simulink model "Controle_velocidade"  (R2021a)
settings: Solver=VariableStepAuto  StartTime=0.0  StopTime=10.0  RelTol=1e-3
values from neighbouring files (symbols this model uses):
  B = 0    [P1_script.m]    (also in simulacao1.m)
  J = 0.001    [P1_script.m]    (also in simulacao1.m = 0.00252)
  Kac = 1/Kpc    (= 0.0936205547599)    [P1_script.m]
  Kas = 1/Kps    (= 0.676014937262)    [P1_script.m]
  Kic = Ra*2*pi*Wcc    (= 1633.62817987)    [P1_script.m]
  Kis = J*(2*pi*Wcs)^2/(5*Kt)    (= 185.888948923)    [P1_script.m]
  Kpc = La*2*pi*Wcc    (= 10.6814150222)    [P1_script.m]
  Kps = J*2*pi*Wcs/Kt    (= 1.47925725436)    [P1_script.m]
  Kt = Te_rated/Ia_rated    (= 0.424752712124)    [P1_script.m]    (also in simulacao1.m)
  La = 1.7e-3    (= 0.0017)    [P1_script.m]    (also in simulacao1.m)
  Ra = 0.26    [P1_script.m]    (also in simulacao1.m)
settings Model: Creator=taylo  LastModifiedBy=taylo

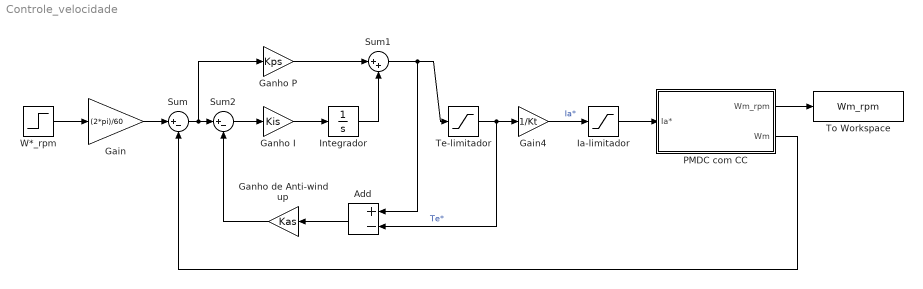
== system Controle_velocidade ==
  Add : Sum  Inputs=+-
  Gain : Gain  Gain=(2*pi)/60
  Gain4 : Gain  Gain=1/Kt
  Ganho I : Gain  Gain=Kis
  Ganho P : Gain  Gain=Kps
  Ganho de Anti-wind up : Gain  Gain=Kas
  Ia-limitador : Saturate
  Integrador : Integrator
  PMDC com CC : Subsystem
  Sum : Sum  Inputs=|+-
  Sum1 : Sum  Inputs=|++
  Sum2 : Sum  Inputs=|+-
  Te-limitador : Saturate
  To Workspace : ToWorkspace  VariableName=Wm_rpm  SaveFormat=Timeseries  SampleTime=-1
  W*_rpm : Step  SampleTime=0
  wires:
  Gain/1 -> Sum/1
  Integrador/1 -> Sum1/2
  Ganho P/1 -> Sum1/1
  Sum1/1 -> Add/1, Te-limitador/1
  Ganho I/1 -> Integrador/1
  Te-limitador/1 -> Add/2, Gain4/1  "Te*"
  Gain4/1 -> Ia-limitador/1  "Ia*"
  Ia-limitador/1 -> PMDC com CC/1(Ia*)
  Sum/1 -> Ganho P/1, Sum2/1
  Sum2/1 -> Ganho I/1
  Add/1 -> Ganho de Anti-wind up/1
  Ganho de Anti-wind up/1 -> Sum2/2
  W*_rpm/1 -> Gain/1
  PMDC com CC/1(Wm_rpm) -> To Workspace/1
  PMDC com CC/2(Wm) -> Sum/2

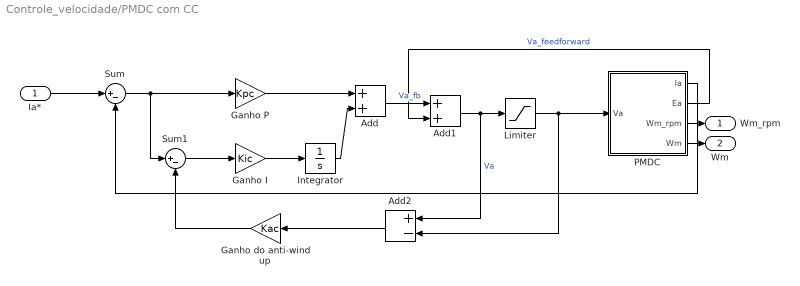
== system Controle_velocidade/PMDC com CC ==
  Ia* : Inport
  Add : Sum
  Add1 : Sum
  Add2 : Sum  Inputs=+-
  Ganho I : Gain  Gain=Kic
  Ganho P : Gain  Gain=Kpc
  Ganho do anti-wind up : Gain  Gain=Kac
  Integrator : Integrator
  Limiter : Saturate
  PMDC : Subsystem
  Sum : Sum  Inputs=|+-
  Sum1 : Sum  Inputs=|+-
  Wm_rpm : Outport
  Wm : Outport  Port=2
  wires:
  Sum/1 -> Sum1/1, Ganho P/1
  Integrator/1 -> Add/2
  Add1/1 -> Add2/1, Limiter/1  "Va"
  Limiter/1 -> Add2/2, PMDC/1(Va)
  Ganho P/1 -> Add/1
  PMDC/1(Ia) -> Sum/2
  Sum1/1 -> Ganho I/1
  Ganho do anti-wind up/1 -> Sum1/2
  Add2/1 -> Ganho do anti-wind up/1
  PMDC/2(Ea) -> Add1/2  "Va_feedforward"
  Add/1 -> Add1/1  "Va_fb"
  Ganho I/1 -> Integrator/1
  Ia*/1 -> Sum/1
  PMDC/4(Wm) -> Wm/1
  PMDC/3(Wm_rpm) -> Wm_rpm/1

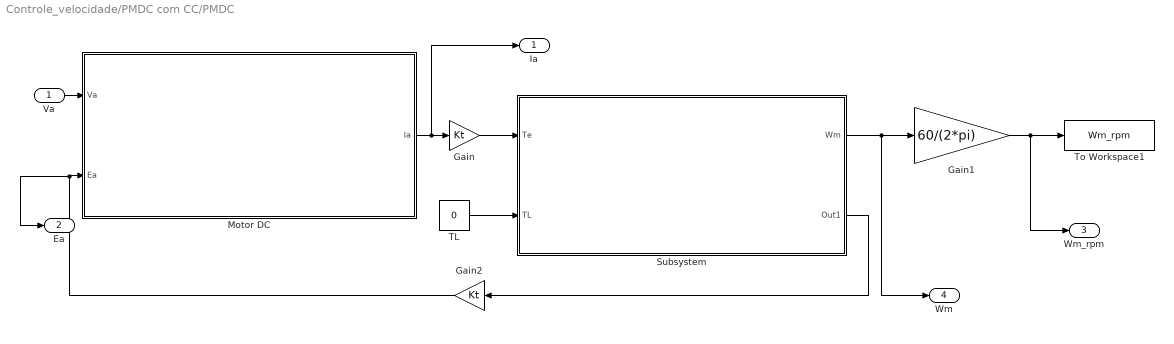
== system Controle_velocidade/PMDC com CC/PMDC ==
  Va : Inport
  Gain : Gain  Gain=Kt
  Gain1 : Gain  Gain=60/(2*pi)
  Gain2 : Gain  Gain=Kt
  Motor DC : Subsystem
  Subsystem : Subsystem
  TL : Constant  Value=0
  To Workspace1 : ToWorkspace  VariableName=Wm_rpm  SaveFormat=Timeseries  SampleTime=-1
  Ia : Outport
  Ea : Outport  Port=2
  Wm_rpm : Outport  Port=3
  Wm : Outport  Port=4
  wires:
  Motor DC/1(Ia) -> Ia/1, Gain/1
  Gain2/1 -> Ea/1, Motor DC/2(Ea)
  Gain/1 -> Subsystem/1(Te)
  Subsystem/1(Wm) -> Wm/1, Gain1/1
  Subsystem/2(Out1) -> Gain2/1
  TL/1 -> Subsystem/2(TL)
  Gain1/1 -> Wm_rpm/1, To Workspace1/1
  Va/1 -> Motor DC/1(Va)

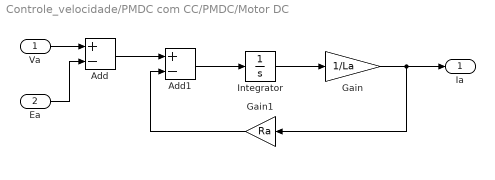
== system Controle_velocidade/PMDC com CC/PMDC/Motor DC ==
  Va : Inport
  Ea : Inport  Port=2
  Add : Sum  Inputs=+-
  Add1 : Sum  Inputs=+-
  Gain : Gain  Gain=1/La
  Gain1 : Gain  Gain=Ra
  Integrator : Integrator
  Ia : Outport
  wires:
  Add1/1 -> Integrator/1
  Gain1/1 -> Add1/2
  Add/1 -> Add1/1
  Va/1 -> Add/1
  Integrator/1 -> Gain/1
  Ea/1 -> Add/2
  Gain/1 -> Gain1/1, Ia/1

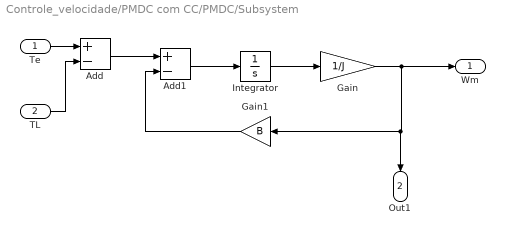
== system Controle_velocidade/PMDC com CC/PMDC/Subsystem ==
  Te : Inport
  TL : Inport  Port=2
  Add : Sum  Inputs=+-
  Add1 : Sum  Inputs=+-
  Gain : Gain  Gain=1/J
  Gain1 : Gain  Gain=B
  Integrator : Integrator
  Wm : Outport
  Out1 : Outport  Port=2
  wires:
  Te/1 -> Add/1
  Gain/1 -> Wm/1, Out1/1, Gain1/1
  Add/1 -> Add1/1
  TL/1 -> Add/2
  Add1/1 -> Integrator/1
  Gain1/1 -> Add1/2
  Integrator/1 -> Gain/1
